simulink model "PID_WindUp_Lab2"  (R2020a)
settings: Solver=VariableStepAuto  StartTime=0.0  StopTime=20  RelTol=1e-3
model workspace (MAT data in the model file):
  Kd = Simulink.Parameter
  Kd.Value = 0.0008954
  Kd.DataType = 'auto'
  Kd.Dimensions = [1 1]
  Ki = Simulink.Parameter
  Ki.Value = 0.39
  Ki.DataType = 'auto'
  Ki.Dimensions = [1 1]
  Kp = Simulink.Parameter
  Kp.Value = 0.0121
  Kp.DataType = 'auto'
  Kp.Dimensions = [1 1]
  Ts = Simulink.Parameter
  Ts.Value = 0.01
  Ts.DataType = 'auto'
  Ts.Dimensions = [1 1]
undefined symbols (not defined in the file): DiscIntNeverNeededParam
libraries: simulink x1
settings Model: Creator=Lenovo  LastModifiedBy=Lenovo
settings OptimizationCC: DefaultParameterBehavior=Inlined  EnhancedBackFolding=on  PassReuseOutputArgsAs=Individual arguments  ZeroExternalMemoryAtStartup=off  ZeroInternalMemoryAtStartup=off  OptimizeBlockOrder=speed  DifferentSizesBufferReuse=on  OptimizationCustomize=off  EfficientTunableParamExpr=on
settings DebuggingCC: ParameterTunabilityLossMsg=error
settings SFSimCC: MATLABDynamicMemAlloc=off
settings RTWCC: SystemTargetFile=ert.tlc  TemplateMakefile=ert_default_tmf
settings CodeAppCC: ForceParamTrailComments=on  IgnoreCustomStorageClasses=off  OperatorAnnotations=on  SimulinkDataObjDesc=on  SFDataObjDesc=on  InsertBlockDesc=on
settings ERTTargetCC: TargetLangStandard=C99 (ISO)  GenerateSampleERTMain=on  InlinedParameterPlacement=NonHierarchical  ERTCustomFileTemplate=example_file_process.tlc

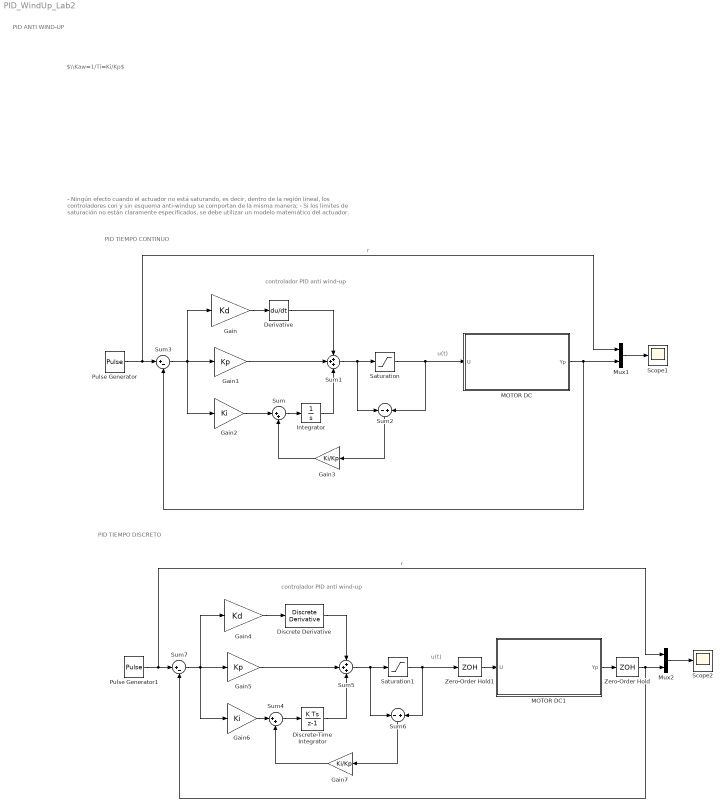
== system PID_WindUp_Lab2 ==
  note: PID TIEMPO CONTINUO
  note: controlador PID anti wind-up
  note: u(t)
  note: - Ningún efecto cuando el actuador no está saturando, es decir, dentro de la región lineal, los controladores con y sin esquema anti-windup
      | se comportan de la misma manera;
      | - Si los límites de saturación no están claramente especificados, se debe utilizar un modelo matemático del actuador.
  note: $\\Kaw=1/Ti=Ki/Kp$
  note: PID ANTI WIND-UP
  note: controlador PID anti wind-up
  note: u(t)
  note: PID TIEMPO DISCRETO
  Derivative : Derivative
  Discrete Derivative : simulink/Discrete/Discrete Derivative  gainval=1.0  ICPrevScaledInput=0.0  OutMin=[]  OutMax=[]  OutDataType=fixdt(1, 16)  OutScaling=2^-10  DoSatur=off
  Discrete-Time Integrator : DiscreteIntegrator  SampleTime=Ts  ICPrevOutput=DiscIntNeverNeededParam  ICPrevScaledInput=DiscIntNeverNeededParam
  Gain : Gain  Gain=Kd
  Gain1 : Gain  Gain=Kp
  Gain2 : Gain  Gain=Ki
  Gain3 : Gain  Gain=Ki/Kp
  Gain4 : Gain  Gain=Kd
  Gain5 : Gain  Gain=Kp
  Gain6 : Gain  Gain=Ki
  Gain7 : Gain  Gain=Ki/Kp
  Integrator : Integrator
  MOTOR DC : Subsystem
  MOTOR DC1 : Subsystem
  Mux1 : Mux  Inputs=2
  Mux2 : Mux  Inputs=2
  Pulse Generator : DiscretePulseGenerator  PulseType=Time based  Amplitude=3.14  Period=10  PulseWidth=50
  Pulse Generator1 : DiscretePulseGenerator  PulseType=Time based  Amplitude=3.14  Period=10  PulseWidth=50
  Saturation : Saturate  UpperLimit=17  LowerLimit=0
  Saturation1 : Saturate  UpperLimit=17  LowerLimit=0
  Scope1 : Scope
  Scope2 : Scope
  Sum : Sum  Inputs=|++
  Sum1 : Sum  Inputs=+++
  Sum2 : Sum  Inputs=-+
  Sum3 : Sum  Inputs=|+-
  Sum4 : Sum  Inputs=|++
  Sum5 : Sum  Inputs=+++
  Sum6 : Sum  Inputs=-+
  Sum7 : Sum  Inputs=|+-
  Zero-Order Hold : ZeroOrderHold  SampleTime=Ts
  Zero-Order Hold1 : ZeroOrderHold  SampleTime=Ts
  wires:
  Gain/1 -> Derivative/1
  Gain2/1 -> Sum/1
  Derivative/1 -> Sum1/1
  Gain1/1 -> Sum1/2
  Sum/1 -> Integrator/1
  Integrator/1 -> Sum1/3
  Gain3/1 -> Sum/2
  Sum1/1 -> Sum2/1, Saturation/1
  Saturation/1 -> MOTOR DC/1(U), Sum2/2
  Sum2/1 -> Gain3/1
  Pulse Generator/1 -> Mux1/1, Sum3/1  "r"
  Sum3/1 -> Gain2/1, Gain/1, Gain1/1
  MOTOR DC/1(Yp) -> Mux1/2, Sum3/2
  Mux1/1 -> Scope1/1
  Mux2/1 -> Scope2/1
  Saturation1/1 -> Zero-Order Hold1/1, Sum6/2
  Discrete Derivative/1 -> Sum5/1
  Gain7/1 -> Sum4/2
  Gain6/1 -> Sum4/1
  Sum5/1 -> Sum6/1, Saturation1/1
  Pulse Generator1/1 -> Mux2/1, Sum7/1  "r"
  Gain5/1 -> Sum5/2
  Sum6/1 -> Gain7/1
  Discrete-Time Integrator/1 -> Sum5/3
  Gain4/1 -> Discrete Derivative/1
  Sum4/1 -> Discrete-Time Integrator/1
  Sum7/1 -> Gain6/1, Gain4/1, Gain5/1
  MOTOR DC1/1(Yp) -> Zero-Order Hold/1
  Zero-Order Hold/1 -> Sum7/2, Mux2/2
  Zero-Order Hold1/1 -> MOTOR DC1/1(U)

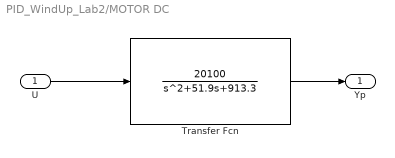
== system PID_WindUp_Lab2/MOTOR DC ==
  U : Inport
  Transfer Fcn : TransferFcn  Numerator=[20100]  Denominator="[1   51.9  913.3]"
  Yp : Outport
  wires:
  Transfer Fcn/1 -> Yp/1
  U/1 -> Transfer Fcn/1

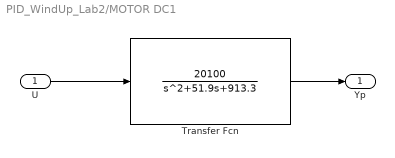
== system PID_WindUp_Lab2/MOTOR DC1 ==
  U : Inport
  Transfer Fcn : TransferFcn  Numerator=[20100]  Denominator="[1   51.9  913.3]"
  Yp : Outport
  wires:
  Transfer Fcn/1 -> Yp/1
  U/1 -> Transfer Fcn/1
